simulink library "pathGeometry_ul"  (R2018b)
settings: Solver=VariableStepAuto  StartTime=0.0  StopTime=10.0  RelTol=1e-3
undefined symbols (not defined in the file or in its folder): initializeVariantsFromBlock
settings Model: Creator=mcobb  LastModifiedBy=jldanie5

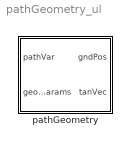
== system pathGeometry_ul ==
  pathGeometry : Subsystem  LoadFcn=initializeVariantsFromBlock(gcb)  InitFcn=initializeVariantsFromBlock(gcb)  StartFcn=initializeVariantsFromBlock(gcb)  Variant=on

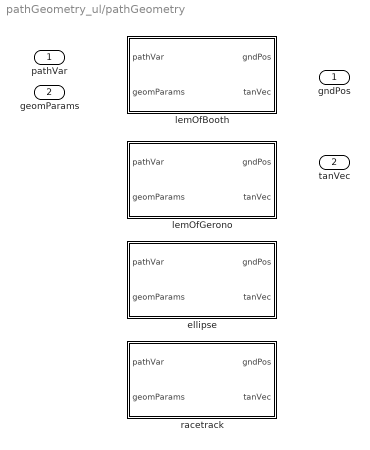
== system pathGeometry_ul/pathGeometry ==
  pathVar : Inport
  geomParams : Inport  Port=2
  ellipse : MATLAB Function  TreatAsAtomicUnit=on  VariantControl=VSS_pathGeometry_ellipse
  lemOfBooth : MATLAB Function  TreatAsAtomicUnit=on  VariantControl=VSS_pathGeometry_lemOfBooth
  lemOfGerono : MATLAB Function  TreatAsAtomicUnit=on  VariantControl=VSS_pathGeometry_lemOfGerono
  racetrack : MATLAB Function  TreatAsAtomicUnit=on  VariantControl=VSS_pathGeometry_racetrack
  gndPos : Outport
  tanVec : Outport  Port=2

== matlab function pathGeometry_ul/pathGeometry/lemOfGerono ==
  data: pathVar input; gndPos output; geomParams input; tanVec output
function [gndPos,tanVec] = fcn(pathVar,geomParams)
[gndPos,tanVec] = lemOfGerono(pathVar,geomParams);

== matlab function pathGeometry_ul/pathGeometry/lemOfBooth ==
  data: pathVar input; gndPos output; geomParams input; tanVec output
function [gndPos,tanVec] = fcn(pathVar,geomParams)
[gndPos,tanVec] = lemOfBooth(pathVar,geomParams);

== matlab function pathGeometry_ul/pathGeometry/ellipse ==
  data: pathVar input; gndPos output; geomParams input; tanVec output
function [gndPos,tanVec] = fcn(pathVar,geomParams)
[gndPos,tanVec] = ellipse(pathVar,geomParams);

== matlab function pathGeometry_ul/pathGeometry/racetrack ==
  data: pathVar input; gndPos output; geomParams input; tanVec output
function [gndPos,tanVec] = fcn(pathVar,geomParams)
[gndPos,tanVec] = racetrack(pathVar,geomParams);
